simulink model "quad_plant"  (R2025b)
settings: Solver=ode4  StartTime=0.0  StopTime=3  FixedStep=0.01  RelTol=1e-3
undefined symbols (not defined in the file): g, Ixx, Iyy, Izz, kQ, kT, l, lambda, m
settings Model: Creator=ONGC  LastModifiedBy=ONGC

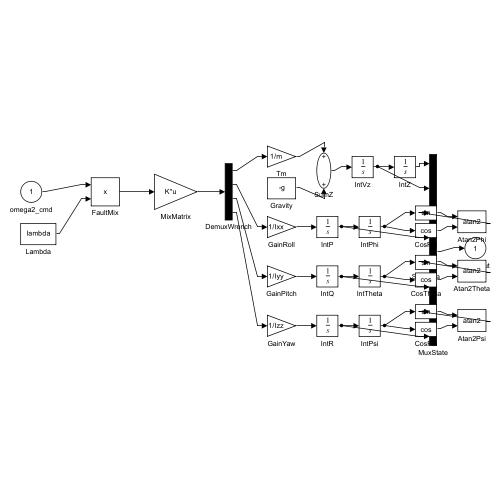
[thumbnail: Simulink's stored preview of the top-level diagram]
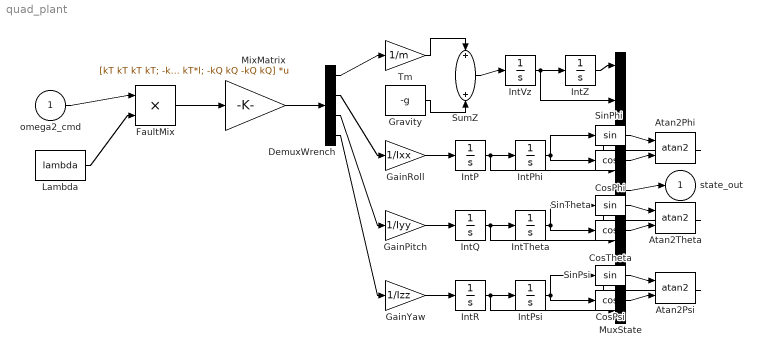
== system quad_plant ==
  omega2_cmd : Inport  PortDimensions=4
  Atan2Phi : Trigonometry  Operator=atan2
  Atan2Psi : Trigonometry  Operator=atan2
  Atan2Theta : Trigonometry  Operator=atan2
  CosPhi : Trigonometry  Operator=cos
  CosPsi : Trigonometry  Operator=cos
  CosTheta : Trigonometry  Operator=cos
  DemuxWrench : Demux
  FaultMix : Product  Inputs=**
  GainPitch : Gain  Gain=1/Iyy
  GainRoll : Gain  Gain=1/Ixx
  GainYaw : Gain  Gain=1/Izz
  Gravity : Constant  Value=-g
  IntP : Integrator
  IntPhi : Integrator
  IntPsi : Integrator
  IntQ : Integrator
  IntR : Integrator
  IntTheta : Integrator
  IntVz : Integrator
  IntZ : Integrator  InitialCondition=1
  Lambda : Constant  Value=lambda
  MixMatrix : Gain  Gain=[kT kT kT kT; -kT*l kT*l kT*l -kT*l; -kT*l -kT*l kT*l kT*l; -kQ kQ -kQ kQ]  Multiplication=Matrix(K*u)
  MuxState : Mux  Inputs=8
  SinPhi : Trigonometry
  SinPsi : Trigonometry
  SinTheta : Trigonometry
  SumZ : Sum
  Tm : Gain  Gain=1/m
  state_out : Outport
  wires:
  omega2_cmd/1 -> FaultMix/1
  Lambda/1 -> FaultMix/2
  FaultMix/1 -> MixMatrix/1
  MixMatrix/1 -> DemuxWrench/1
  DemuxWrench/1 -> Tm/1
  Tm/1 -> SumZ/1
  Gravity/1 -> SumZ/2
  SumZ/1 -> IntVz/1
  IntVz/1 -> IntZ/1, MuxState/2
  DemuxWrench/2 -> GainRoll/1
  GainRoll/1 -> IntP/1
  IntP/1 -> IntPhi/1, MuxState/4
  DemuxWrench/3 -> GainPitch/1
  GainPitch/1 -> IntQ/1
  IntQ/1 -> IntTheta/1, MuxState/6
  DemuxWrench/4 -> GainYaw/1
  GainYaw/1 -> IntR/1
  IntR/1 -> IntPsi/1, MuxState/8
  IntZ/1 -> MuxState/1
  MuxState/1 -> state_out/1
  IntPhi/1 -> SinPhi/1, CosPhi/1
  SinPhi/1 -> Atan2Phi/1
  CosPhi/1 -> Atan2Phi/2
  Atan2Phi/1 -> MuxState/3
  IntTheta/1 -> SinTheta/1, CosTheta/1
  SinTheta/1 -> Atan2Theta/1
  CosTheta/1 -> Atan2Theta/2
  Atan2Theta/1 -> MuxState/5
  IntPsi/1 -> SinPsi/1, CosPsi/1
  SinPsi/1 -> Atan2Psi/1
  CosPsi/1 -> Atan2Psi/2
  Atan2Psi/1 -> MuxState/7
